simulink model "deltino"  (R2021b)
settings: Solver=VariableStepAuto  StartTime=0.0  StopTime=inf  FixedStep=0.0001  RelTol=1e-3
values from neighbouring files (symbols this model uses):
  alpha1 = 0    [compute_deltino_dyn_parallel.m]
  alpha2 = 2/3*pi    (= 2.09439510239)    [compute_deltino_dyn_parallel.m]
  alpha3 = 4/3*pi    (= 4.18879020479)    [compute_deltino_dyn_parallel.m]
  H = 0.05    [main.m]
  J_T = [J_1', J_2', J_3', J_4']    [main.m]
  K_d = 10    [main.m]
  K_el = 10000    [main.m]
  K_i = 1    [main.m]
  K_p = 200    [main.m]
  K_v = 10    [main.m]
  mu = 0.8    [main.m]
  ni_0 = zeros(18,1)    [main.m]
  offset1 = [l1/2; l2/2; -h/2]    [compute_deltino_dyn_parallel.m]    (also in main.m = [+l1/2; +l2/2; -h/2])
  offset2 = [l1/2; -l2/2; -h/2]    [compute_deltino_dyn_parallel.m]    (also in main.m = [+l1/2; -l2/2; -h/2])
  offset3 = [-l1/2; -l2/2; -h/2]    [compute_deltino_dyn_parallel.m]    (also in main.m)
  offset4 = [-l1/2; l2/2; -h/2]    [compute_deltino_dyn_parallel.m]    (also in main.m = [-l1/2; +l2/2; -h/2])
  p_leg1_0 = forward_kin(theta_leg1_0)    [main.m]
  p_leg2_0 = forward_kin(theta_leg2_0)    [main.m]
  p_leg3_0 = forward_kin(theta_leg3_0)    [main.m]
  p_leg4_0 = forward_kin(theta_leg4_0)    [main.m]
  points_ccw = [+0.1,  0.00 ... (first row only)    [main.m]
  points_cw = [-0.1,  0.00 ... (first row only)    [main.m]
  q_0 = [base_0; ypr_0; theta_leg1_0; ee_leg1_0; theta_leg2_0; ee_leg2_0;        theta_leg3_0; ee_leg3_0; theta_leg4_0; ee_leg4_0;]    [main.m]
  ratio = 2    [main.m]
  steps = 4+2*ratio    (= 8)    [main.m]
  theta_leg1_0 = [pi/6; pi/6; pi/6]    [main.m]
  theta_leg2_0 = [pi/6; pi/6; pi/6]    [main.m]
  theta_leg3_0 = [pi/6; pi/6; pi/6]    [main.m]
  theta_leg4_0 = [pi/6; pi/6; pi/6]    [main.m]
  ts = T/steps    (= 0.1875)    [main.m]
  ts2 = 3*ts    (= 0.5625)    [main.m]
  vel = 0.2    [main.m]
undefined symbols (not defined in the file or in its folder): l1, l_A, l_B, R, radius0, radius1, radius2, theta, WPs
libraries: simulink x14, dspsigops x12
(part 1 of 10)
settings Model: PacingRate=0.280000  Creator=alber  LastModifiedBy=albertomarianobili
settings SolverCC: AlgebraicLoopSolver=TrustRegion

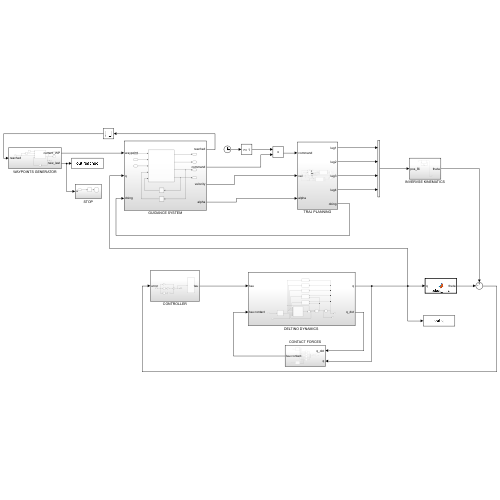
[thumbnail: Simulink's stored preview of the top-level diagram]
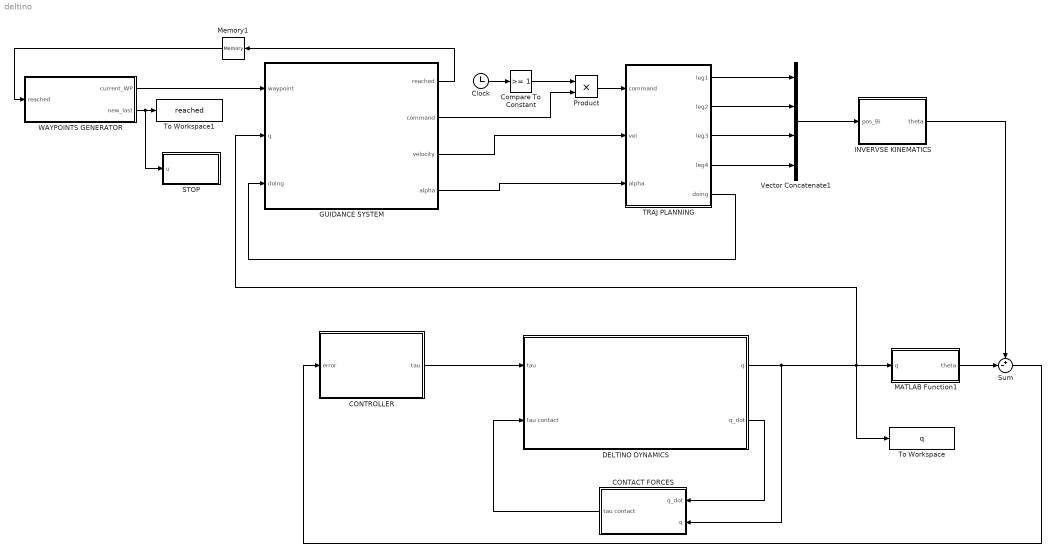
== system deltino ==
  CONTACT FORCES : Subsystem
  CONTROLLER : Subsystem
  Clock : Clock
  Compare To Constant : simulink/Logic and Bit Operations/Compare To Constant  relop=>=  const=1  OutDataTypeStr=boolean
  "DELTINO DYNAMICS " : Subsystem
  GUIDANCE SYSTEM : Subsystem
  INVERVSE KINEMATICS : Subsystem
  MATLAB Function1 : MATLAB Function  TreatAsAtomicUnit=on
  Memory1 : Memory
  Product : Product
  STOP : Subsystem
  Sum : Sum  Inputs=+-|
  TRAJ PLANNING : Subsystem
  To Workspace : ToWorkspace  VariableName=q  SaveFormat=Timeseries  SampleTime=-1
  To Workspace1 : ToWorkspace  VariableName=reached  SaveFormat=Timeseries  SampleTime=-1
  Vector Concatenate1 : Concatenate  NumInputs=4  Mode=Multidimensional array
  WAYPOINTS GENERATOR : Subsystem
  wires:
  CONTROLLER/1(tau) -> "DELTINO DYNAMICS "/1(tau)
  Sum/1 -> CONTROLLER/1(error)
  TRAJ PLANNING/2(leg2) -> Vector Concatenate1/2
  TRAJ PLANNING/1(leg1) -> Vector Concatenate1/1
  TRAJ PLANNING/4(leg4) -> Vector Concatenate1/4
  TRAJ PLANNING/3(leg3) -> Vector Concatenate1/3
  GUIDANCE SYSTEM/4(alpha) -> TRAJ PLANNING/3(alpha)
  MATLAB Function1/1(theta) -> Sum/2
  GUIDANCE SYSTEM/1(reached) -> Memory1/1
  WAYPOINTS GENERATOR/1(current_WP) -> GUIDANCE SYSTEM/1(waypoint)
  Memory1/1 -> WAYPOINTS GENERATOR/1(reached)
  "DELTINO DYNAMICS "/1(q) -> CONTACT FORCES/2(q), GUIDANCE SYSTEM/2(q), MATLAB Function1/1(q), To Workspace/1
  TRAJ PLANNING/5(doing) -> GUIDANCE SYSTEM/3(doing)
  GUIDANCE SYSTEM/2(command) -> Product/2
  GUIDANCE SYSTEM/3(velocity) -> TRAJ PLANNING/2(vel)
  Clock/1 -> Compare To Constant/1
  Compare To Constant/1 -> Product/1
  Product/1 -> TRAJ PLANNING/1(command)
  WAYPOINTS GENERATOR/2(new_last) -> STOP/1(u), To Workspace1/1
  Vector Concatenate1/1 -> INVERVSE KINEMATICS/1(pos_Bi)
  INVERVSE KINEMATICS/1(theta) -> Sum/1
  "DELTINO DYNAMICS "/2(q_dot) -> CONTACT FORCES/1(q_dot)
  CONTACT FORCES/1(tau contact) -> "DELTINO DYNAMICS "/2(tau contact)

== system deltino/CONTACT FORCES ==
  q_dot : Inport
  q : Inport  Port=2
  Constant2 : Constant  Value=J_T
  Contact Forces Leg1 : Subsystem
  Contact Forces Leg2 : Subsystem
  Contact Forces Leg3 : Subsystem
  Contact Forces Leg4 : Subsystem
  MATLAB Function1 : MATLAB Function  TreatAsAtomicUnit=on
  MATLAB Function3 : MATLAB Function  TreatAsAtomicUnit=on
  MatrixMultiply : Product  Multiplication=Matrix(*)
  Mux : Mux
  tau contact : Outport
  wires:
  Mux/1 -> MatrixMultiply/2
  MATLAB Function1/4(ee_leg4) -> Contact Forces Leg4/1(p_ee)
  MATLAB Function3/2(ee_dot_leg2) -> Contact Forces Leg2/2(v_ee)
  MATLAB Function1/2(ee_leg2) -> Contact Forces Leg2/1(p_ee)
  MATLAB Function1/3(ee_leg3) -> Contact Forces Leg3/1(p_ee)
  Contact Forces Leg2/1(f) -> Mux/2
  Contact Forces Leg4/1(f) -> Mux/4
  MATLAB Function1/1(ee_leg1) -> Contact Forces Leg1/1(p_ee)
  Contact Forces Leg1/1(f) -> Mux/1
  MATLAB Function3/4(ee_dot_leg4) -> Contact Forces Leg4/2(v_ee)
  MATLAB Function3/1(ee_dot_leg1) -> Contact Forces Leg1/2(v_ee)
  Constant2/1 -> MatrixMultiply/1
  q_dot/1 -> MATLAB Function3/1(q_dot)
  MATLAB Function3/3(ee_dot_leg3) -> Contact Forces Leg3/2(v_ee)
  Contact Forces Leg3/1(f) -> Mux/3
  MatrixMultiply/1 -> tau contact/1
  q/1 -> MATLAB Function1/1(q)

== system deltino/CONTROLLER ==
  error : Inport
  Derivative : Derivative  CoefficientInTFapproximation=50
  Display : Display
  Gain : Gain  Gain=K_d
  Gain1 : Gain  Gain=K_p
  Gain2 : Gain  Gain=K_i
  Integrator : Integrator
  Sum : Sum  Inputs=+++
  tau : Outport
  wires:
  error/1 -> Derivative/1, Gain1/1, Integrator/1
  Integrator/1 -> Gain2/1
  Derivative/1 -> Gain/1
  Gain2/1 -> Sum/2
  Gain1/1 -> Sum/1
  Gain/1 -> Sum/3
  Sum/1 -> Display/1, tau/1

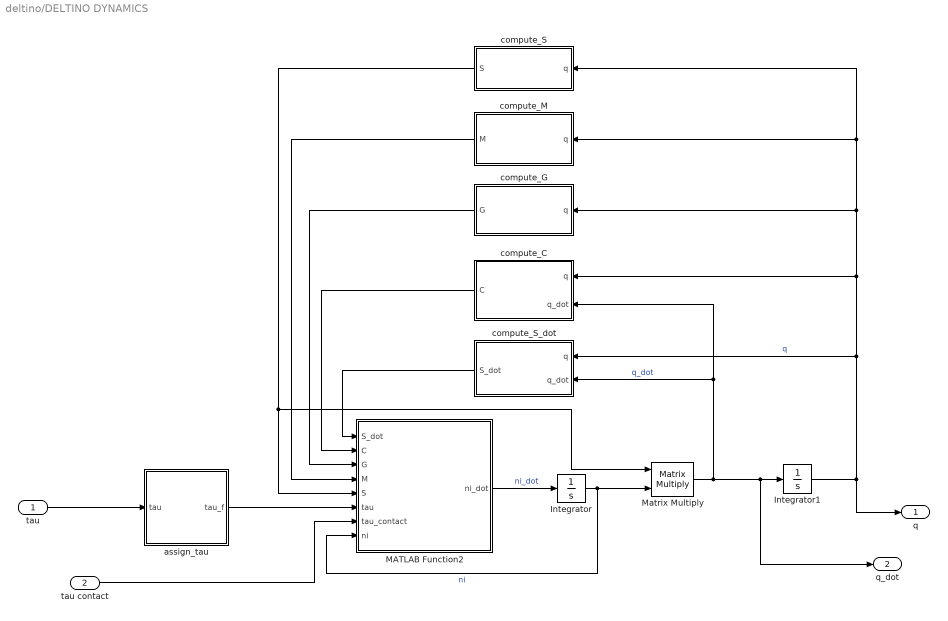
== system deltino/DELTINO DYNAMICS  ==
  tau : Inport
  tau contact : Inport  Port=2
  Integrator : Integrator  InitialCondition=ni_0
  Integrator1 : Integrator  InitialCondition=q_0
  MATLAB Function2 : MATLAB Function  TreatAsAtomicUnit=on
  Matrix Multiply : Product  Multiplication=Matrix(*)
  assign_tau : MATLAB Function  TreatAsAtomicUnit=on
  compute_C : MATLAB Function  TreatAsAtomicUnit=on
  compute_G : MATLAB Function  TreatAsAtomicUnit=on
  compute_M : MATLAB Function  TreatAsAtomicUnit=on
  compute_S : MATLAB Function  TreatAsAtomicUnit=on
  compute_S_dot : MATLAB Function  TreatAsAtomicUnit=on
  q : Outport
  q_dot : Outport  Port=2
  wires:
  Integrator1/1 -> q/1, compute_M/1(q), compute_S/1(q), compute_G/1(q), compute_C/1(q), compute_S_dot/1(q)  "q"
  Matrix Multiply/1 -> compute_C/2(q_dot), compute_S_dot/2(q_dot), q_dot/1, Integrator1/1  "q_dot"
  Integrator/1 -> Matrix Multiply/2, MATLAB Function2/8(ni)  "ni"
  compute_S_dot/1(S_dot) -> MATLAB Function2/1(S_dot)
  compute_M/1(M) -> MATLAB Function2/4(M)
  compute_S/1(S) -> Matrix Multiply/1, MATLAB Function2/5(S)
  MATLAB Function2/1(ni_dot) -> Integrator/1  "ni_dot"
  tau/1 -> assign_tau/1(tau)
  compute_C/1(C) -> MATLAB Function2/2(C)
  compute_G/1(G) -> MATLAB Function2/3(G)
  assign_tau/1(tau_f) -> MATLAB Function2/6(tau)
  tau contact/1 -> MATLAB Function2/7(tau_contact)

== system deltino/GUIDANCE SYSTEM ==
  waypoint : Inport
  q : Inport  Port=2
  doing : Inport  Port=3
  MATLAB Function : MATLAB Function  TreatAsAtomicUnit=on
  Memory : Memory
  Memory1 : Memory
  reached : Outport
  command : Outport  Port=2
  velocity : Outport  Port=3
  alpha : Outport  Port=4
  wires:
  MATLAB Function/4(alpha) -> alpha/1, Memory1/1
  MATLAB Function/2(mode) -> command/1
  waypoint/1 -> MATLAB Function/1(wp)
  q/1 -> MATLAB Function/2(q)
  MATLAB Function/3(velocity) -> velocity/1, Memory/1
  MATLAB Function/1(reached) -> reached/1
  doing/1 -> MATLAB Function/3(doing)
  Memory1/1 -> MATLAB Function/5(old_alpha)
  Memory/1 -> MATLAB Function/4(old_vel)

== system deltino/INVERVSE KINEMATICS ==
  pos_Bi : Inport
  Memory : Memory  InitialCondition=[theta_leg1_0; theta_leg2_0; theta_leg3_0; theta_leg4_0]
  Pos_to_Theta : MATLAB Function  TreatAsAtomicUnit=on
  theta : Outport
  wires:
  Pos_to_Theta/2(theta_old) -> Memory/1
  Memory/1 -> Pos_to_Theta/2("theta_old ")
  pos_Bi/1 -> Pos_to_Theta/1(pos_Bi)
  Pos_to_Theta/1(theta) -> theta/1

== system deltino/STOP ==
  u : Inport
  Compare To Constant1 : simulink/Logic and Bit Operations/Compare To Constant  relop=>=  const=4  OutDataTypeStr=boolean
  Stop Simulation : Stop
  wires:
  Compare To Constant1/1 -> Stop Simulation/1
  u/1 -> Compare To Constant1/1

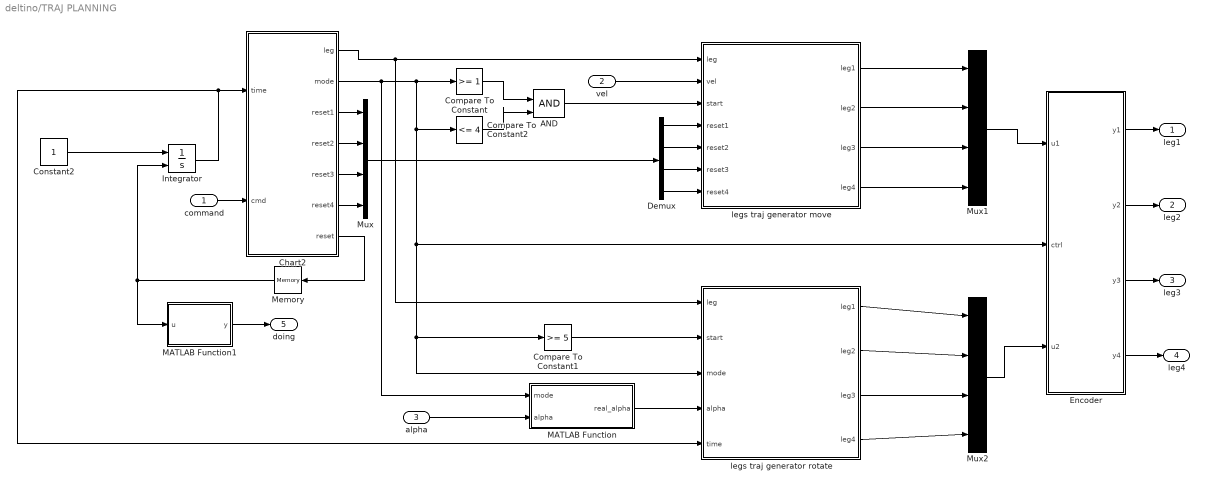
== system deltino/TRAJ PLANNING ==
  command : Inport
  vel : Inport  Port=2
  alpha : Inport  Port=3
  " Encoder" : MATLAB Function  TreatAsAtomicUnit=on
  AND : Logic  IconShape=distinctive  AllPortsSameDT=off  OutDataTypeStr=boolean
  Chart2 : Stateflow chart  TreatAsAtomicUnit=on
      settings: PortSchema="{\"entries\":[{\"content\":{\"sides\":[{\"content\":{\"connectorIds\":[\"In1\",\"In2\"]},\"type\":\"ConnectorPlacement.EquallySpacedRectSide\",\"uuid\":\"1e0c41a3-cebd-41cb-8a93-7a7bf92eebf6\"},{\"content\":{\"connectorIds\":[\"Out2\",\"Out3\",\"Out4\",\"Out5\",\"Out6\",\"Out7\",\"Out1\"],\"side\":\"RIGHT\"},\"type\":\"ConnectorPlacement.EquallySpacedRectSide\",\"uuid\":\"6e8626e0-42cb-4e6c-b1bb-c4d6db9bdd55\"},{\"content\":{\"connectorIds\":[],\"side\":\"TOP\"},\"type\":\"ConnectorPlacement.EquallySpacedRectSide\",\"uuid\":\"3bbd30af-d298-4b5b-952b-a7c5a39acad1\"}]},\"type\":\"ConnectorPlacement.EquallySpacedConnector\",\"uuid\":\"6b50d4a5-2ed0-4cfe-bea9-ec2e14be68f9\"}],\"packageUris\":[\"http://schema.mathworks.com/mf0/Connector/R2020b\"],\"version\":\"1.0\"}"
  Compare To Constant : simulink/Logic and Bit Operations/Compare To Constant  relop=>=  const=1  OutDataTypeStr=boolean
  Compare To Constant1 : simulink/Logic and Bit Operations/Compare To Constant  relop=>=  const=5  OutDataTypeStr=boolean
  Compare To Constant2 : simulink/Logic and Bit Operations/Compare To Constant  relop=<=  const=4  OutDataTypeStr=boolean
  Constant2 : Constant
  Demux : Demux
  Integrator : Integrator  ExternalReset=level
  MATLAB Function : MATLAB Function  TreatAsAtomicUnit=on
  MATLAB Function1 : MATLAB Function  TreatAsAtomicUnit=on
  Memory : Memory  InitialCondition=1
  Mux : Mux
  Mux1 : Mux
  Mux2 : Mux
  legs traj generator move : Subsystem
  legs traj generator rotate : Subsystem
  leg1 : Outport
  leg2 : Outport  Port=2
  leg3 : Outport  Port=3
  leg4 : Outport  Port=4
  doing : Outport  Port=5
  wires:
  Constant2/1 -> Integrator/1
  Integrator/1 -> Chart2/1(time), legs traj generator rotate/5(time)
  command/1 -> Chart2/2(cmd)
  Chart2/1(reset) -> Memory/1
  Memory/1 -> Integrator/2, MATLAB Function1/1(u)
  legs traj generator move/2(leg2) -> Mux1/2
  legs traj generator move/1(leg1) -> Mux1/1
  legs traj generator move/3(leg3) -> Mux1/3
  legs traj generator move/4(leg4) -> Mux1/4
  " Encoder"/1(y1) -> leg1/1
  " Encoder"/2(y2) -> leg2/1
  " Encoder"/3(y3) -> leg3/1
  " Encoder"/4(y4) -> leg4/1
  Mux1/1 -> " Encoder"/1(u1)
  Chart2/3(mode) -> MATLAB Function/1(mode), " Encoder"/2(ctrl), legs traj generator rotate/3(mode), Compare To Constant1/1, Compare To Constant2/1, Compare To Constant/1
  Chart2/2(leg) -> legs traj generator rotate/1(leg), legs traj generator move/1(leg)
  legs traj generator rotate/1(leg1) -> Mux2/1
  legs traj generator rotate/2(leg2) -> Mux2/2
  legs traj generator rotate/3(leg3) -> Mux2/3
  legs traj generator rotate/4(leg4) -> Mux2/4
  Mux2/1 -> " Encoder"/3(u2)
  Compare To Constant1/1 -> legs traj generator rotate/2(start)
  Compare To Constant/1 -> AND/1
  Compare To Constant2/1 -> AND/2
  AND/1 -> legs traj generator move/3(start)
  MATLAB Function/1(real_alpha) -> legs traj generator rotate/4(alpha)
  MATLAB Function1/1(y) -> doing/1
  vel/1 -> legs traj generator move/2(vel)
  alpha/1 -> MATLAB Function/2(alpha)
  Chart2/4(reset1) -> Mux/1
  Chart2/7(reset4) -> Mux/4
  Chart2/6(reset3) -> Mux/3
  Chart2/5(reset2) -> Mux/2
  Demux/4 -> legs traj generator move/7(reset4)
  Mux/1 -> Demux/1
  Demux/1 -> legs traj generator move/4(reset1)
  Demux/2 -> legs traj generator move/5(reset2)
  Demux/3 -> legs traj generator move/6(reset3)

== system deltino/WAYPOINTS GENERATOR ==
  reached : Inport
  Constant : Constant  Value=WPs
  MATLAB Function : MATLAB Function  TreatAsAtomicUnit=on
  Memory1 : Memory  InitialCondition=1
  Memory2 : Memory
  Scope1 : Scope
  current_WP : Outport
  new_last : Outport  Port=2
  wires:
  MATLAB Function/2(new_last) -> Memory1/1, new_last/1
  Memory1/1 -> MATLAB Function/4(old_last)
  reached/1 -> MATLAB Function/3(reached), Memory2/1  "reached"
  Constant/1 -> MATLAB Function/1(all_WPs)
  Memory2/1 -> MATLAB Function/2(old_reached)  "old_reached"
  MATLAB Function/1(current_WP) -> Scope1/1, current_WP/1

== system deltino/CONTACT FORCES/Contact Forces Leg1 ==
  p_ee : Inport
  v_ee : Inport  Port=2
  Contact Forces : MATLAB Function  TreatAsAtomicUnit=on
  Memory : Memory  InitialCondition=[0;0]
  Memory1 : Memory
  f : Outport
  wires:
  Memory1/1 -> Contact Forces/3("contact ")
  Contact Forces/3(p0) -> Memory/1
  p_ee/1 -> Contact Forces/1(p_ee)
  v_ee/1 -> Contact Forces/2(v_ee)
  Contact Forces/2(contact) -> Memory1/1
  Memory/1 -> Contact Forces/4("p0 ")
  Contact Forces/1(f) -> f/1

== system deltino/CONTACT FORCES/Contact Forces Leg2 ==
  p_ee : Inport
  v_ee : Inport  Port=2
  Contact Forces : MATLAB Function  TreatAsAtomicUnit=on
  Memory : Memory  InitialCondition=[0;0]
  Memory1 : Memory
  f : Outport
  wires:
  Memory1/1 -> Contact Forces/3("contact ")
  Contact Forces/3(p0) -> Memory/1
  p_ee/1 -> Contact Forces/1(p_ee)
  v_ee/1 -> Contact Forces/2(v_ee)
  Contact Forces/2(contact) -> Memory1/1
  Memory/1 -> Contact Forces/4("p0 ")
  Contact Forces/1(f) -> f/1

== system deltino/CONTACT FORCES/Contact Forces Leg3 ==
  p_ee : Inport
  v_ee : Inport  Port=2
  Contact Forces : MATLAB Function  TreatAsAtomicUnit=on
  Memory : Memory  InitialCondition=[0;0]
  Memory1 : Memory
  f : Outport
  wires:
  Memory1/1 -> Contact Forces/3("contact ")
  Contact Forces/3(p0) -> Memory/1
  p_ee/1 -> Contact Forces/1(p_ee)
  v_ee/1 -> Contact Forces/2(v_ee)
  Contact Forces/2(contact) -> Memory1/1
  Memory/1 -> Contact Forces/4("p0 ")
  Contact Forces/1(f) -> f/1

== system deltino/CONTACT FORCES/Contact Forces Leg4 ==
  p_ee : Inport
  v_ee : Inport  Port=2
  Contact Forces : MATLAB Function  TreatAsAtomicUnit=on
  Memory : Memory  InitialCondition=[0;0]
  Memory1 : Memory
  f : Outport
  wires:
  Memory1/1 -> Contact Forces/3("contact ")
  Contact Forces/3(p0) -> Memory/1
  p_ee/1 -> Contact Forces/1(p_ee)
  v_ee/1 -> Contact Forces/2(v_ee)
  Contact Forces/2(contact) -> Memory1/1
  Memory/1 -> Contact Forces/4("p0 ")
  Contact Forces/1(f) -> f/1

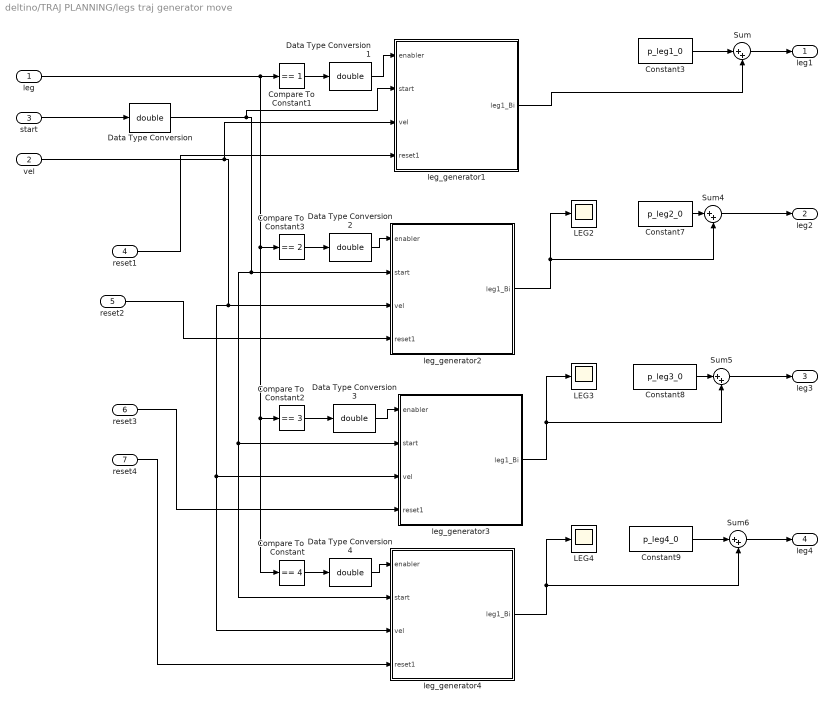
== system deltino/TRAJ PLANNING/legs traj generator move ==
  leg : Inport
  vel : Inport  Port=2
  start : Inport  Port=3
  reset1 : Inport  Port=4
  reset2 : Inport  Port=5
  reset3 : Inport  Port=6
  reset4 : Inport  Port=7
  Compare To Constant : simulink/Logic and Bit Operations/Compare To Constant  relop===  const=4  OutDataTypeStr=boolean
  Compare To Constant1 : simulink/Logic and Bit Operations/Compare To Constant  relop===  const=1  OutDataTypeStr=boolean
  Compare To Constant2 : simulink/Logic and Bit Operations/Compare To Constant  relop===  const=3  OutDataTypeStr=boolean
  Compare To Constant3 : simulink/Logic and Bit Operations/Compare To Constant  relop===  const=2  OutDataTypeStr=boolean
  Constant3 : Constant  Value=p_leg1_0
  Constant7 : Constant  Value=p_leg2_0
  Constant8 : Constant  Value=p_leg3_0
  Constant9 : Constant  Value=p_leg4_0
  Data Type Conversion{,1..4} (5 alike) : DataTypeConversion  OutDataTypeStr=double
  LEG2 : Scope
  LEG3 : Scope
  LEG4 : Scope
  Sum{,4..6} (4 alike) : Sum  Inputs=|++
  leg_generator1 : Subsystem
  leg_generator2 : Subsystem
  leg_generator3 : Subsystem
  leg_generator4 : Subsystem
  leg1 : Outport
  leg2 : Outport  Port=2
  leg3 : Outport  Port=3
  leg4 : Outport  Port=4
  wires:
  Constant7/1 -> Sum4/1
  leg_generator1/1(leg1_Bi) -> Sum/2
  leg_generator4/1(leg1_Bi) -> Sum6/2, LEG4/1
  Sum6/1 -> leg4/1
  start/1 -> Data Type Conversion/1
  Sum/1 -> leg1/1
  Compare To Constant3/1 -> Data Type Conversion2/1
  leg_generator3/1(leg1_Bi) -> LEG3/1, Sum5/2
  Compare To Constant1/1 -> Data Type Conversion1/1
  Sum5/1 -> leg3/1
  leg/1 -> Compare To Constant3/1, Compare To Constant/1, Compare To Constant2/1, Compare To Constant1/1
  leg_generator2/1(leg1_Bi) -> LEG2/1, Sum4/2
  Compare To Constant2/1 -> Data Type Conversion3/1
  Compare To Constant/1 -> Data Type Conversion4/1
  Sum4/1 -> leg2/1
  Constant3/1 -> Sum/1
  Constant8/1 -> Sum5/1
  Constant9/1 -> Sum6/1
  Data Type Conversion/1 -> leg_generator1/2(start), leg_generator2/2(start), leg_generator3/2(start), leg_generator4/2(start)
  Data Type Conversion1/1 -> leg_generator1/1(enabler)
  Data Type Conversion2/1 -> leg_generator2/1(enabler)
  Data Type Conversion3/1 -> leg_generator3/1(enabler)
  Data Type Conversion4/1 -> leg_generator4/1(enabler)
  vel/1 -> leg_generator1/3(vel), leg_generator2/3(vel), leg_generator3/3(vel), leg_generator4/3(vel)
  reset1/1 -> leg_generator1/4(reset1)
  reset2/1 -> leg_generator2/4(reset1)
  reset3/1 -> leg_generator3/4(reset1)
  reset4/1 -> leg_generator4/4(reset1)

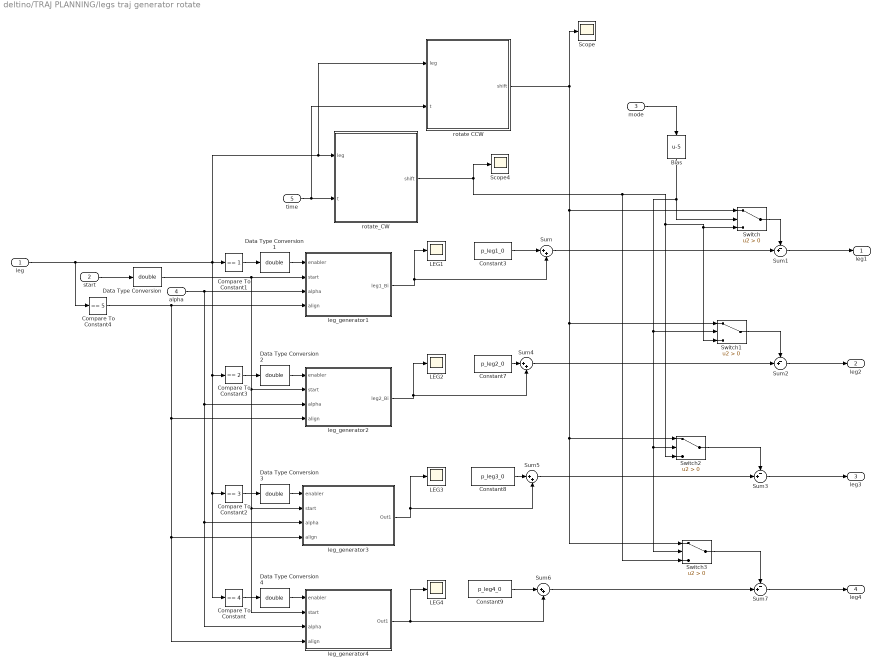
== system deltino/TRAJ PLANNING/legs traj generator rotate ==
  leg : Inport
  start : Inport  Port=2
  mode : Inport  Port=3
  alpha : Inport  Port=4
  time : Inport  Port=5
  Bias : Bias  Bias=-5
  Compare To Constant : simulink/Logic and Bit Operations/Compare To Constant  relop===  const=4  OutDataTypeStr=boolean
  Compare To Constant1 : simulink/Logic and Bit Operations/Compare To Constant  relop===  const=1  OutDataTypeStr=boolean
  Compare To Constant2 : simulink/Logic and Bit Operations/Compare To Constant  relop===  const=3  OutDataTypeStr=boolean
  Compare To Constant3 : simulink/Logic and Bit Operations/Compare To Constant  relop===  const=2  OutDataTypeStr=boolean
  Compare To Constant4 : simulink/Logic and Bit Operations/Compare To Constant  relop===  const=5  OutDataTypeStr=boolean
  Constant3 : Constant  Value=p_leg1_0
  Constant7 : Constant  Value=p_leg2_0
  Constant8 : Constant  Value=p_leg3_0
  Constant9 : Constant  Value=p_leg4_0
  Data Type Conversion{,1..4} (5 alike) : DataTypeConversion  OutDataTypeStr=double
  LEG{1..4} (4 alike) : Scope
  Scope : Scope
  Scope4 : Scope
  Sum{,4..6} (4 alike) : Sum  Inputs=|++
  Sum{1..3,7} (4 alike) : Sum  Inputs=-+|
  Switch{,1..3} (4 alike) : Switch  Criteria=u2 > Threshold
  leg_generator1 : Subsystem
  leg_generator2 : Subsystem
  leg_generator3 : Subsystem
  leg_generator4 : Subsystem
  rotate CCW : MATLAB Function  TreatAsAtomicUnit=on
  rotate_CW : MATLAB Function  TreatAsAtomicUnit=on
  leg1 : Outport
  leg2 : Outport  Port=2
  leg3 : Outport  Port=3
  leg4 : Outport  Port=4
  wires:
  Constant7/1 -> Sum4/1
  leg_generator1/1(leg1_Bi) -> Sum/2, LEG1/1
  leg_generator4/1(Out1) -> Sum6/2, LEG4/1
  Sum6/1 -> Sum7/2
  start/1 -> Data Type Conversion/1
  Sum/1 -> Sum1/2
  Compare To Constant3/1 -> Data Type Conversion2/1
  leg_generator3/1(Out1) -> LEG3/1, Sum5/2
  Compare To Constant1/1 -> Data Type Conversion1/1
  Sum5/1 -> Sum3/2
  leg/1 -> rotate_CW/1(leg), rotate CCW/1(leg), Compare To Constant/1, Compare To Constant2/1, Compare To Constant3/1, Compare To Constant1/1, Compare To Constant4/1
  leg_generator2/1(leg2_Bi) -> LEG2/1, Sum4/2
  Compare To Constant2/1 -> Data Type Conversion3/1
  Compare To Constant/1 -> Data Type Conversion4/1
  Sum4/1 -> Sum2/2
  Constant3/1 -> Sum/1
  Constant8/1 -> Sum5/1
  Constant9/1 -> Sum6/1
  Data Type Conversion/1 -> leg_generator1/2(start), leg_generator4/2(start), leg_generator3/2(start), leg_generator2/2(start)
  Data Type Conversion1/1 -> leg_generator1/1(enabler)
  Data Type Conversion2/1 -> leg_generator2/1(enabler)
  Data Type Conversion3/1 -> leg_generator3/1(enabler)
  Data Type Conversion4/1 -> leg_generator4/1(enabler)
  alpha/1 -> leg_generator2/3(alpha), leg_generator4/3(alpha), leg_generator3/3(alpha), leg_generator1/3(alpha)
  Compare To Constant4/1 -> leg_generator4/4(align), leg_generator3/4(align), leg_generator2/4(align), leg_generator1/4(align)
  Sum1/1 -> leg1/1
  Sum7/1 -> leg4/1
  Sum3/1 -> leg3/1
  Sum2/1 -> leg2/1
  time/1 -> rotate_CW/2(t), rotate CCW/2(t)
  rotate_CW/1(shift) -> Scope4/1, Switch3/3, Switch2/3, Switch/3, Switch1/3
  Switch3/1 -> Sum7/1
  Switch2/1 -> Sum3/1
  Switch1/1 -> Sum2/1
  Switch/1 -> Sum1/1
  mode/1 -> Bias/1
  Bias/1 -> Switch/2, Switch1/2, Switch3/2, Switch2/2
  rotate CCW/1(shift) -> Scope/1, Switch2/1, Switch3/1, Switch1/1, Switch/1

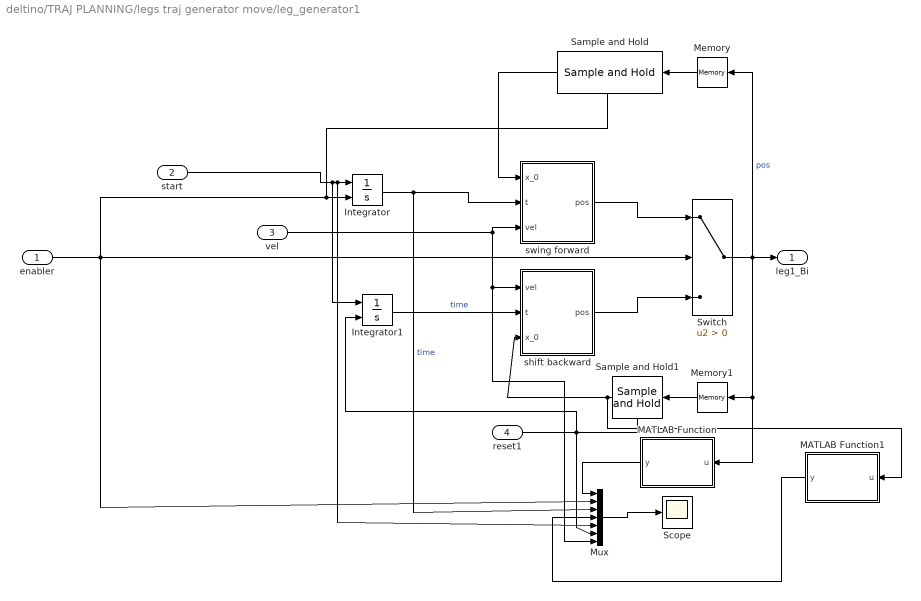
== system deltino/TRAJ PLANNING/legs traj generator move/leg_generator1 ==
  enabler : Inport
  start : Inport  Port=2
  vel : Inport  Port=3
  reset1 : Inport  Port=4
  Integrator : Integrator  ExternalReset=either
  Integrator1 : Integrator  ExternalReset=rising
  MATLAB Function : MATLAB Function  TreatAsAtomicUnit=on
  MATLAB Function1 : MATLAB Function  TreatAsAtomicUnit=on
  Memory : Memory  InitialCondition=[0;0;0]
  Memory1 : Memory  InitialCondition=[0;0;0]
  Mux : Mux  Inputs=7
  Sample and Hold : dspsigops/Sample and Hold  trig=Rising edge  initCond=[0;0;0]  latchinput=off
  Sample and Hold1 : dspsigops/Sample and Hold  trig=Rising edge  initCond=[0;0;0]  latchinput=off
  Scope : Scope
  Switch : Switch  Criteria=u2 > Threshold
  shift backward : MATLAB Function  TreatAsAtomicUnit=on
  swing forward : MATLAB Function  TreatAsAtomicUnit=on
  leg1_Bi : Outport
  wires:
  Switch/1 -> Memory/1, leg1_Bi/1, MATLAB Function/1(u), Memory1/1  "pos"
  shift backward/1(pos) -> Switch/3
  swing forward/1(pos) -> Switch/1
  Integrator/1 -> Mux/3, swing forward/2(t)  "time"
  start/1 -> Integrator1/1, Mux/5, Integrator/1
  Sample and Hold/1 -> swing forward/1(x_0)
  Memory/1 -> Sample and Hold/1
  Mux/1 -> Scope/1
  Memory1/1 -> Sample and Hold1/1
  enabler/1 -> Sample and Hold/Trigger, Integrator/2, Mux/2, Switch/2
  Sample and Hold1/1 -> MATLAB Function1/1(u), shift backward/3(x_0)
  vel/1 -> shift backward/1(vel), Mux/7, swing forward/3(vel)
  MATLAB Function/1(y) -> Mux/1
  MATLAB Function1/1(y) -> Mux/4
  reset1/1 -> Integrator1/2, Sample and Hold1/Trigger, Mux/6
  Integrator1/1 -> shift backward/2(t)  "time"

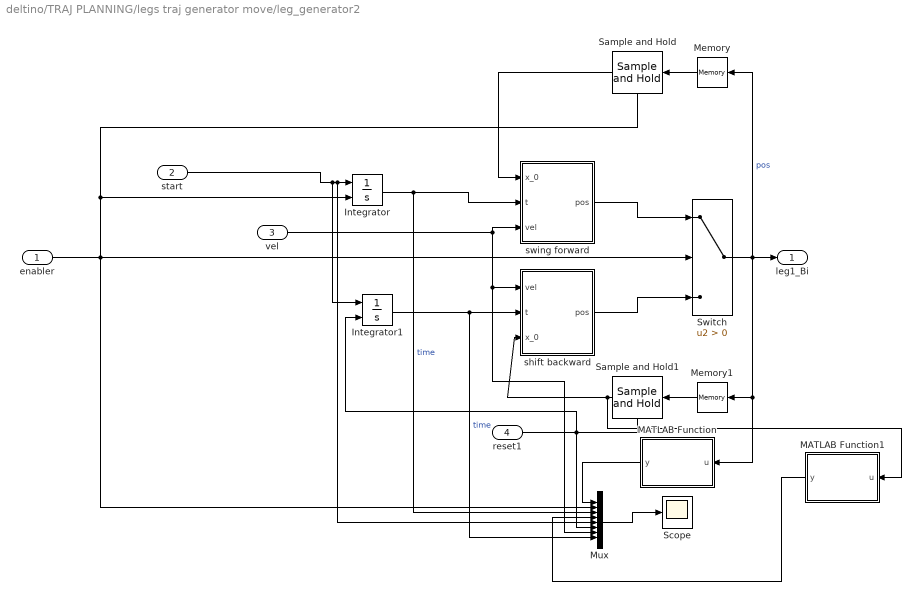
== system deltino/TRAJ PLANNING/legs traj generator move/leg_generator2 ==
  enabler : Inport
  start : Inport  Port=2
  vel : Inport  Port=3
  reset1 : Inport  Port=4
  Integrator : Integrator  ExternalReset=either
  Integrator1 : Integrator  ExternalReset=rising
  MATLAB Function : MATLAB Function  TreatAsAtomicUnit=on
  MATLAB Function1 : MATLAB Function  TreatAsAtomicUnit=on
  Memory : Memory  InitialCondition=[0;0;0]
  Memory1 : Memory  InitialCondition=[0;0;0]
  Mux : Mux  Inputs=8
  Sample and Hold : dspsigops/Sample and Hold  trig=Rising edge  initCond=[0;0;0]  latchinput=off
  Sample and Hold1 : dspsigops/Sample and Hold  trig=Rising edge  initCond=[0;0;0]  latchinput=off
  Scope : Scope
  Switch : Switch  Criteria=u2 > Threshold
  shift backward : MATLAB Function  TreatAsAtomicUnit=on
  swing forward : MATLAB Function  TreatAsAtomicUnit=on
  leg1_Bi : Outport
  wires:
  Switch/1 -> Memory/1, leg1_Bi/1, MATLAB Function/1(u), Memory1/1  "pos"
  shift backward/1(pos) -> Switch/3
  swing forward/1(pos) -> Switch/1
  Integrator/1 -> Mux/3, swing forward/2(t)  "time"
  start/1 -> Integrator1/1, Mux/5, Integrator/1
  Sample and Hold/1 -> swing forward/1(x_0)
  Memory/1 -> Sample and Hold/1
  Mux/1 -> Scope/1
  Memory1/1 -> Sample and Hold1/1
  enabler/1 -> Sample and Hold/Trigger, Integrator/2, Mux/2, Switch/2
  Sample and Hold1/1 -> MATLAB Function1/1(u), shift backward/3(x_0)
  vel/1 -> shift backward/1(vel), Mux/7, swing forward/3(vel)
  MATLAB Function/1(y) -> Mux/1
  MATLAB Function1/1(y) -> Mux/4
  reset1/1 -> Integrator1/2, Sample and Hold1/Trigger, Mux/6
  Integrator1/1 -> Mux/8, shift backward/2(t)  "time"

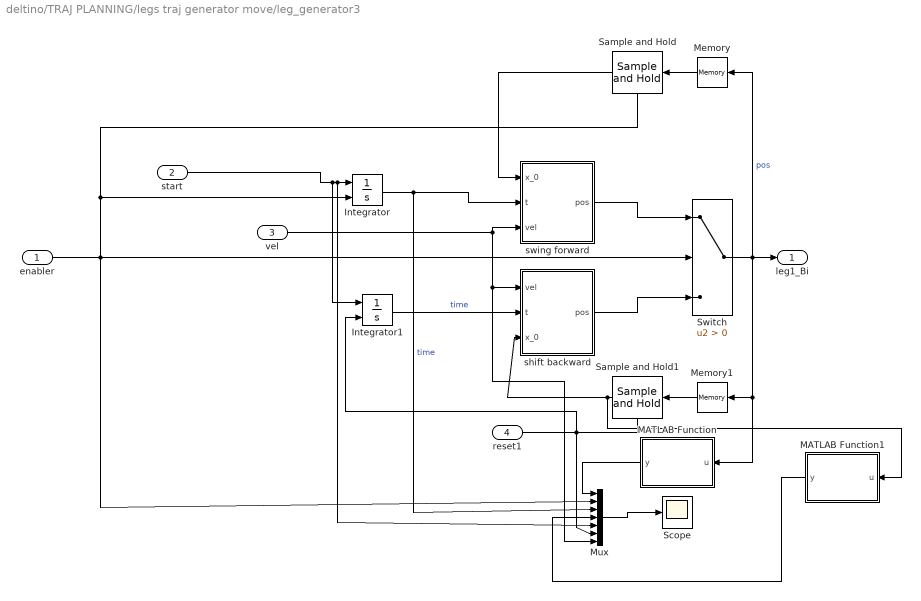
== system deltino/TRAJ PLANNING/legs traj generator move/leg_generator3 ==
  enabler : Inport
  start : Inport  Port=2
  vel : Inport  Port=3
  reset1 : Inport  Port=4
  Integrator : Integrator  ExternalReset=either
  Integrator1 : Integrator  ExternalReset=rising
  MATLAB Function : MATLAB Function  TreatAsAtomicUnit=on
  MATLAB Function1 : MATLAB Function  TreatAsAtomicUnit=on
  Memory : Memory  InitialCondition=[0;0;0]
  Memory1 : Memory  InitialCondition=[0;0;0]
  Mux : Mux  Inputs=7
  Sample and Hold : dspsigops/Sample and Hold  trig=Rising edge  initCond=[0;0;0]  latchinput=off
  Sample and Hold1 : dspsigops/Sample and Hold  trig=Rising edge  initCond=[0;0;0]  latchinput=off
  Scope : Scope
  Switch : Switch  Criteria=u2 > Threshold
  shift backward : MATLAB Function  TreatAsAtomicUnit=on
  swing forward : MATLAB Function  TreatAsAtomicUnit=on
  leg1_Bi : Outport
  wires:
  Switch/1 -> Memory/1, leg1_Bi/1, MATLAB Function/1(u), Memory1/1  "pos"
  shift backward/1(pos) -> Switch/3
  swing forward/1(pos) -> Switch/1
  Integrator/1 -> Mux/3, swing forward/2(t)  "time"
  start/1 -> Integrator1/1, Mux/5, Integrator/1
  Sample and Hold/1 -> swing forward/1(x_0)
  Memory/1 -> Sample and Hold/1
  Mux/1 -> Scope/1
  Memory1/1 -> Sample and Hold1/1
  enabler/1 -> Sample and Hold/Trigger, Integrator/2, Mux/2, Switch/2
  Sample and Hold1/1 -> MATLAB Function1/1(u), shift backward/3(x_0)
  vel/1 -> shift backward/1(vel), Mux/7, swing forward/3(vel)
  MATLAB Function/1(y) -> Mux/1
  MATLAB Function1/1(y) -> Mux/4
  reset1/1 -> Integrator1/2, Sample and Hold1/Trigger, Mux/6
  Integrator1/1 -> shift backward/2(t)  "time"

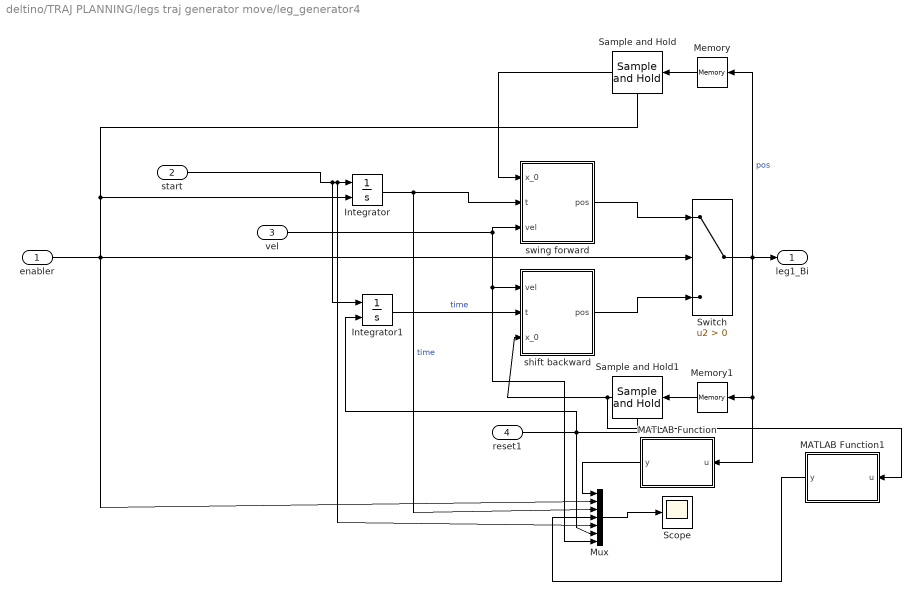
== system deltino/TRAJ PLANNING/legs traj generator move/leg_generator4 ==
  enabler : Inport
  start : Inport  Port=2
  vel : Inport  Port=3
  reset1 : Inport  Port=4
  Integrator : Integrator  ExternalReset=either
  Integrator1 : Integrator  ExternalReset=rising
  MATLAB Function : MATLAB Function  TreatAsAtomicUnit=on
  MATLAB Function1 : MATLAB Function  TreatAsAtomicUnit=on
  Memory : Memory  InitialCondition=[0;0;0]
  Memory1 : Memory  InitialCondition=[0;0;0]
  Mux : Mux  Inputs=7
  Sample and Hold : dspsigops/Sample and Hold  trig=Rising edge  initCond=[0;0;0]  latchinput=off
  Sample and Hold1 : dspsigops/Sample and Hold  trig=Rising edge  initCond=[0;0;0]  latchinput=off
  Scope : Scope
  Switch : Switch  Criteria=u2 > Threshold
  shift backward : MATLAB Function  TreatAsAtomicUnit=on
  swing forward : MATLAB Function  TreatAsAtomicUnit=on
  leg1_Bi : Outport
  wires:
  Switch/1 -> Memory/1, leg1_Bi/1, MATLAB Function/1(u), Memory1/1  "pos"
  shift backward/1(pos) -> Switch/3
  swing forward/1(pos) -> Switch/1
  Integrator/1 -> Mux/3, swing forward/2(t)  "time"
  start/1 -> Integrator1/1, Mux/5, Integrator/1
  Sample and Hold/1 -> swing forward/1(x_0)
  Memory/1 -> Sample and Hold/1
  Mux/1 -> Scope/1
  Memory1/1 -> Sample and Hold1/1
  enabler/1 -> Sample and Hold/Trigger, Integrator/2, Mux/2, Switch/2
  Sample and Hold1/1 -> MATLAB Function1/1(u), shift backward/3(x_0)
  vel/1 -> shift backward/1(vel), Mux/7, swing forward/3(vel)
  MATLAB Function/1(y) -> Mux/1
  MATLAB Function1/1(y) -> Mux/4
  reset1/1 -> Integrator1/2, Sample and Hold1/Trigger, Mux/6
  Integrator1/1 -> shift backward/2(t)  "time"

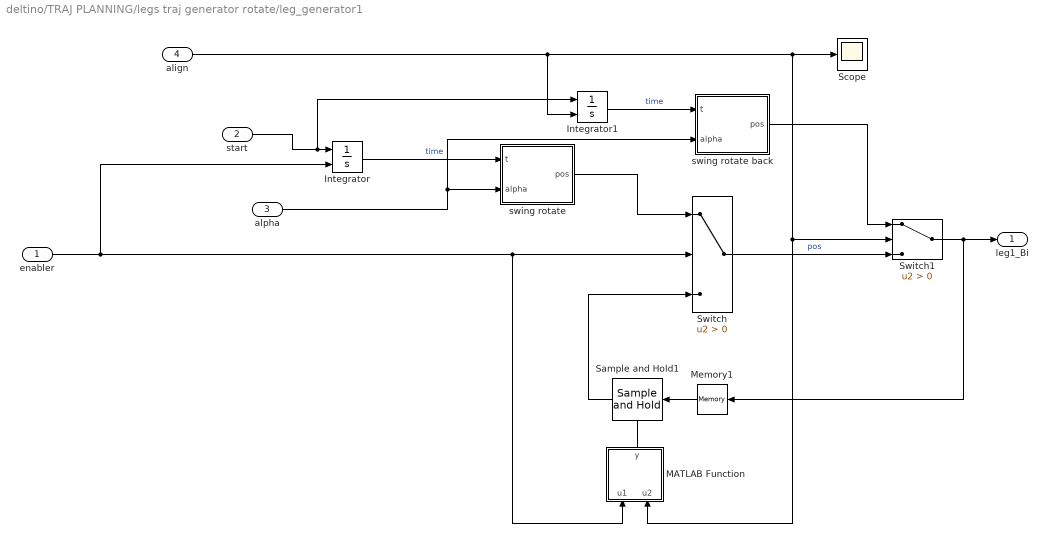
== system deltino/TRAJ PLANNING/legs traj generator rotate/leg_generator1 ==
  enabler : Inport
  start : Inport  Port=2
  alpha : Inport  Port=3
  align : Inport  Port=4
  Integrator : Integrator  ExternalReset=either
  Integrator1 : Integrator  ExternalReset=either
  MATLAB Function : MATLAB Function  TreatAsAtomicUnit=on
  Memory1 : Memory  InitialCondition=[0;0;0]
  Sample and Hold1 : dspsigops/Sample and Hold  trig=Falling edge  initCond=[0;0;0]  latchinput=off
  Scope : Scope
  Switch : Switch  Criteria=u2 > Threshold
  Switch1 : Switch  Criteria=u2 > Threshold
  swing rotate : MATLAB Function  TreatAsAtomicUnit=on
  swing rotate back : MATLAB Function  TreatAsAtomicUnit=on
  leg1_Bi : Outport
  wires:
  Switch/1 -> Switch1/3  "pos"
  swing rotate/1(pos) -> Switch/1
  Integrator/1 -> swing rotate/1(t)  "time"
  start/1 -> Integrator1/1, Integrator/1
  Memory1/1 -> Sample and Hold1/1
  enabler/1 -> MATLAB Function/1(u1), Switch/2, Integrator/2
  Sample and Hold1/1 -> Switch/3
  Switch1/1 -> Memory1/1, leg1_Bi/1
  align/1 -> Scope/1, Switch1/2, MATLAB Function/2(u2), Integrator1/2
  swing rotate back/1(pos) -> Switch1/1
  MATLAB Function/1(y) -> Sample and Hold1/Trigger
  alpha/1 -> swing rotate back/2(alpha), swing rotate/2(alpha)
  Integrator1/1 -> swing rotate back/1(t)  "time"

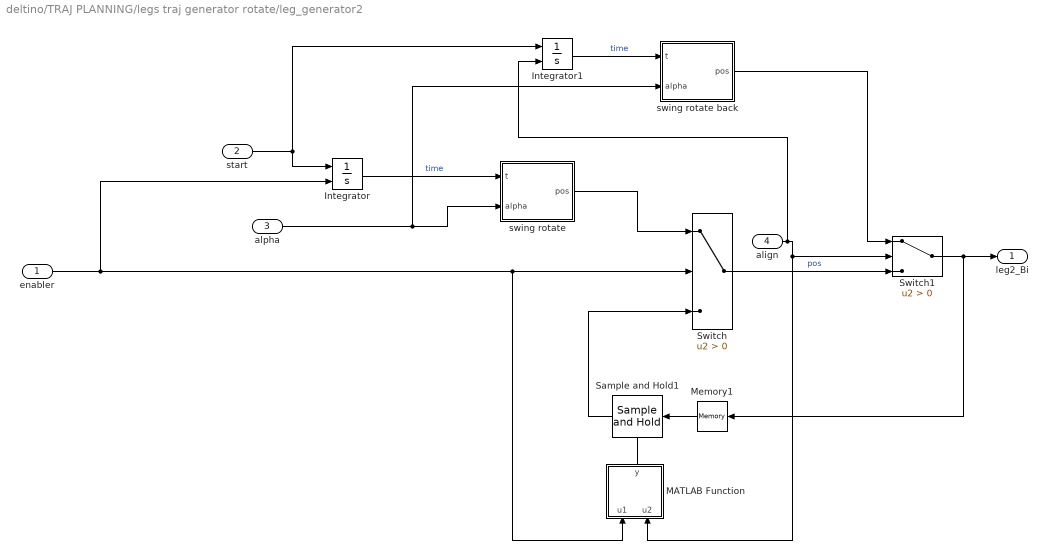
== system deltino/TRAJ PLANNING/legs traj generator rotate/leg_generator2 ==
  enabler : Inport
  start : Inport  Port=2
  alpha : Inport  Port=3
  align : Inport  Port=4
  Integrator : Integrator  ExternalReset=either
  Integrator1 : Integrator  ExternalReset=either
  MATLAB Function : MATLAB Function  TreatAsAtomicUnit=on
  Memory1 : Memory  InitialCondition=[0;0;0]
  Sample and Hold1 : dspsigops/Sample and Hold  trig=Falling edge  initCond=[0;0;0]  latchinput=off
  Switch : Switch  Criteria=u2 > Threshold
  Switch1 : Switch  Criteria=u2 > Threshold
  swing rotate : MATLAB Function  TreatAsAtomicUnit=on
  swing rotate back : MATLAB Function  TreatAsAtomicUnit=on
  leg2_Bi : Outport
  wires:
  Switch/1 -> Switch1/3  "pos"
  swing rotate/1(pos) -> Switch/1
  Integrator/1 -> swing rotate/1(t)  "time"
  start/1 -> Integrator1/1, Integrator/1
  Memory1/1 -> Sample and Hold1/1
  enabler/1 -> MATLAB Function/1(u1), Switch/2, Integrator/2
  Sample and Hold1/1 -> Switch/3
  Switch1/1 -> Memory1/1, leg2_Bi/1
  align/1 -> Integrator1/2, MATLAB Function/2(u2), Switch1/2
  swing rotate back/1(pos) -> Switch1/1
  MATLAB Function/1(y) -> Sample and Hold1/Trigger
  Integrator1/1 -> swing rotate back/1(t)  "time"
  alpha/1 -> swing rotate back/2(alpha), swing rotate/2(alpha)

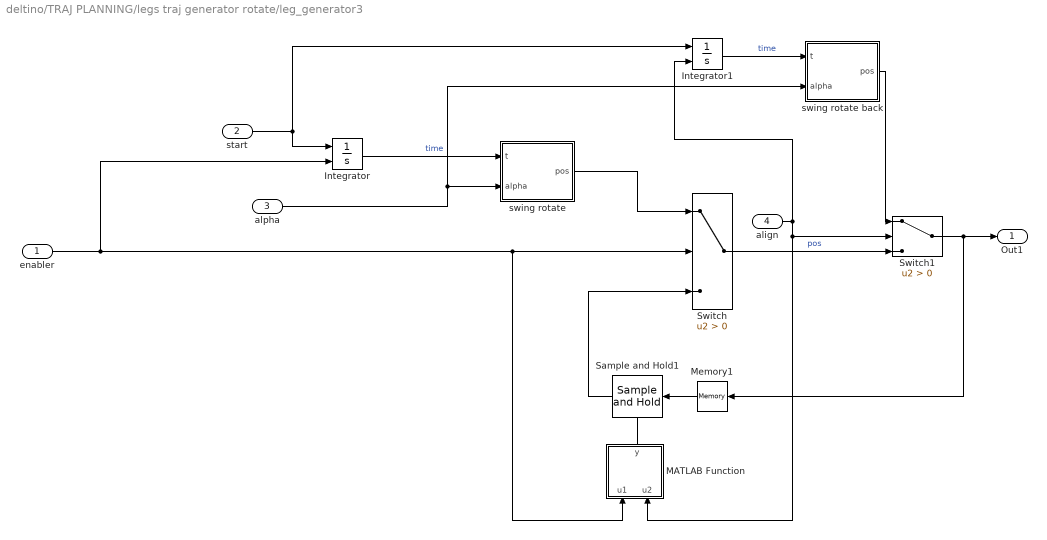
== system deltino/TRAJ PLANNING/legs traj generator rotate/leg_generator3 ==
  enabler : Inport
  start : Inport  Port=2
  alpha : Inport  Port=3
  align : Inport  Port=4
  Integrator : Integrator  ExternalReset=either
  Integrator1 : Integrator  ExternalReset=either
  MATLAB Function : MATLAB Function  TreatAsAtomicUnit=on
  Memory1 : Memory  InitialCondition=[0;0;0]
  Sample and Hold1 : dspsigops/Sample and Hold  trig=Falling edge  initCond=[0;0;0]  latchinput=off
  Switch : Switch  Criteria=u2 > Threshold
  Switch1 : Switch  Criteria=u2 > Threshold
  swing rotate : MATLAB Function  TreatAsAtomicUnit=on
  swing rotate back : MATLAB Function  TreatAsAtomicUnit=on
  Out1 : Outport
  wires:
  Switch/1 -> Switch1/3  "pos"
  swing rotate/1(pos) -> Switch/1
  Integrator/1 -> swing rotate/1(t)  "time"
  start/1 -> Integrator1/1, Integrator/1
  Memory1/1 -> Sample and Hold1/1
  enabler/1 -> MATLAB Function/1(u1), Switch/2, Integrator/2
  Sample and Hold1/1 -> Switch/3
  Switch1/1 -> Memory1/1, Out1/1
  align/1 -> Integrator1/2, MATLAB Function/2(u2), Switch1/2
  swing rotate back/1(pos) -> Switch1/1
  MATLAB Function/1(y) -> Sample and Hold1/Trigger
  alpha/1 -> swing rotate back/2(alpha), swing rotate/2(alpha)
  Integrator1/1 -> swing rotate back/1(t)  "time"

== system deltino/TRAJ PLANNING/legs traj generator rotate/leg_generator4 ==
  enabler : Inport
  start : Inport  Port=2
  alpha : Inport  Port=3
  align : Inport  Port=4
  Integrator : Integrator  ExternalReset=either
  Integrator1 : Integrator  ExternalReset=either
  MATLAB Function : MATLAB Function  TreatAsAtomicUnit=on
  Memory1 : Memory  InitialCondition=[0;0;0]
  Sample and Hold1 : dspsigops/Sample and Hold  trig=Falling edge  initCond=[0;0;0]  latchinput=off
  Switch : Switch  Criteria=u2 > Threshold
  Switch1 : Switch  Criteria=u2 > Threshold
  swing rotate : MATLAB Function  TreatAsAtomicUnit=on
  swing rotate back : MATLAB Function  TreatAsAtomicUnit=on
  Out1 : Outport
  wires:
  Switch/1 -> Switch1/3  "pos"
  swing rotate/1(pos) -> Switch/1
  Integrator/1 -> swing rotate/1(t)  "time"
  start/1 -> Integrator1/1, Integrator/1
  Memory1/1 -> Sample and Hold1/1
  enabler/1 -> MATLAB Function/1(u1), Switch/2, Integrator/2
  Sample and Hold1/1 -> Switch/3
  Switch1/1 -> Memory1/1, Out1/1
  align/1 -> MATLAB Function/2(u2), Integrator1/2, Switch1/2
  MATLAB Function/1(y) -> Sample and Hold1/Trigger
  Integrator1/1 -> swing rotate back/1(t)  "time"
  alpha/1 -> swing rotate back/2(alpha), swing rotate/2(alpha)
  swing rotate back/1(pos) -> Switch1/1
